simulink model "pothole_test"  (R2025a)
settings: Solver=VariableStepAuto  StartTime=0.0  StopTime=10.0  RelTol=1e-3
model workspace (MAT data in the model file):
  vehicle_car = Simulink.Parameter
  vehicle_car.Complexity = 'real'
  vehicle_car.Dimensions = [0 0]
  vehicle_car.DataType = 'auto'
undefined symbols (not defined in the file or in its folder): Defined, Ego, Lane, User
libraries: roadrunnerscenario x4
settings Model: Creator=Shreyas Hegde  LastModifiedBy=Shreyas Hegde

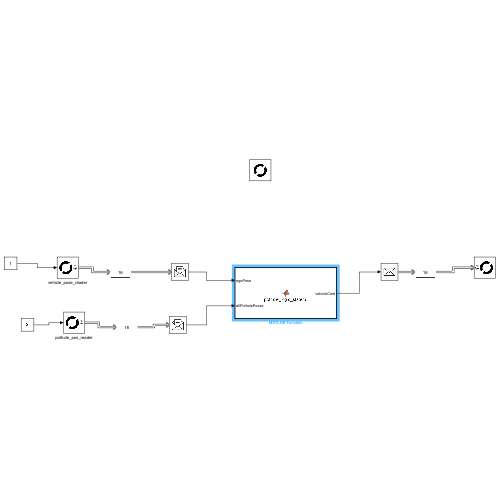
[thumbnail: Simulink's stored preview of the top-level diagram]
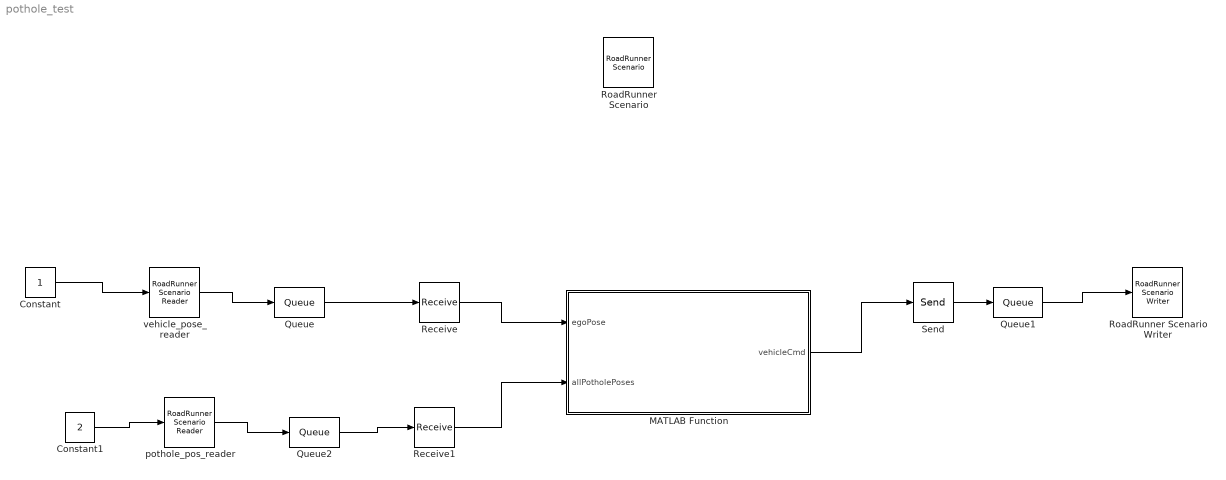
== system pothole_test ==
  Constant : Constant
  Constant1 : Constant  Value=2
  MATLAB Function : MATLAB Function  TreatAsAtomicUnit=on
  Queue : Queue  InputPortMessageModes=m  OutputPortMessageModes=m  OverwriteOldest=on  Capacity=16  QueueType=LIFO
  Queue1 : Queue  InputPortMessageModes=m  OutputPortMessageModes=m  OverwriteOldest=on  Capacity=16  QueueType=LIFO
  Queue2 : Queue  InputPortMessageModes=m  OutputPortMessageModes=m  OverwriteOldest=on  Capacity=16  QueueType=LIFO
  Receive : Receive  InputPortMessageModes=m  UseInternalQueue=off  QueueOverwriting=on  QueueLength=1  QueueType=LIFO
  Receive1 : Receive  InputPortMessageModes=m  UseInternalQueue=off  QueueOverwriting=on  QueueLength=1  QueueType=LIFO
  RoadRunner Scenario : roadrunnerscenario/RoadRunner Scenario  UserDefinedActions={}  UserDefinedEvents={}  PathPoints=500
  RoadRunner Scenario Writer : roadrunnerscenario/RoadRunner Scenario Writer  TopicCategory=Actor  ActorCategory=All Types  EventType=Action Complete  UserDefinedEvent=Event1  VehicleType=Vehicle Pose  TopicType=Actor Pose
  Send : Send  OutputPortMessageModes=m
  pothole_pos_reader : roadrunnerscenario/RoadRunner Scenario Reader  TopicCategory=Actor  ActorCategory=All Types  ActionType=Path Following  EventType=User-Defined  TopicType=Actor Pose  VehicleType=Vehicle Specifications  TrafficSignalType=Traffic Signal Specifications  TrafficSignalControllerType=Traffic Signal Controller Specifications  UserDefinedAction=Action1  UserDefinedEvent=Event1  Filter=Actor ID (provided by input)  AdditionalRelationship=None  SensorTopic=Target Poses  LaneBoundaryOutputTopic=Ego-Lane  SensorID=1  SampleTime=0
  vehicle_pose_reader : roadrunnerscenario/RoadRunner Scenario Reader  TopicCategory=Actor  ActorCategory=All Types  ActionType=Path Following  EventType=User-Defined  TopicType=Actor Pose  VehicleType=Vehicle Specifications  TrafficSignalType=Traffic Signal Specifications  TrafficSignalControllerType=Traffic Signal Controller Specifications  UserDefinedAction=Action1  UserDefinedEvent=Event1  Filter=Actor ID (provided by input)  AdditionalRelationship=None  SensorTopic=Target Poses  LaneBoundaryOutputTopic=Ego-Lane  SensorID=1  SampleTime=0
  wires:
  vehicle_pose_reader/1 -> Queue/1
  Queue/1 -> Receive/1
  Send/1 -> Queue1/1
  Queue1/1 -> RoadRunner Scenario Writer/1
  pothole_pos_reader/1 -> Queue2/1
  Queue2/1 -> Receive1/1
  Receive/1 -> MATLAB Function/1(egoPose)
  Receive1/1 -> MATLAB Function/2(allPotholePoses)
  MATLAB Function/1(vehicleCmd) -> Send/1
  Constant/1 -> vehicle_pose_reader/1
  Constant1/1 -> pothole_pos_reader/1

== matlab function pothole_test/MATLAB Function ==
  data: egoPose input; vehicleCmd output; allPotholePoses input
function vehicleCmd = pothole_logic_stateful(egoPose, allPotholePoses)
% This function uses persistent variables to continuously track the next
% pothole and command the vehicle speed.

% --- Tunable Parameters ---
CRUISING_SPEED = 15;  % m/s (approx 54 km/h)
POTHOLE_SPEED = 5;    % m/s (approx 18 km/h)
ACTION_DISTANCE = 50; % meters

% Use a persistent variable to store the ID of the current target pothole.
persistent targetPotholeID;
if isempty(targetPotholeID)
    targetPotholeID = -1; % Initialize on the first run
end

% Initialize the output command bus to tell Simulink the data type
vehicleCmd = Simulink.Bus.createMATLABStruct('slBusActorCommand');
vehicleCmd.ActorName = "vehicle_car"; % Command is always for our car
vehicleCmd.TargetSpeed = CRUISING_SPEED; % Default to cruising speed

% Exit early if the simulation hasn't provided valid actor data yet
if isempty(egoPose) || egoPose.ActorID == 0
    return;
end

% --- State Machine Logic ---

% 1. Find a new target if we don't currently have one.
if targetPotholeID == -1
    targetPotholeID = findNextPothole(egoPose, allPotholePoses.Poses, -1);
end

% If we still can't find a target (e.g., no potholes left), just cruise.
if targetPotholeID == -1
    return;
end

% 2. Get the current position of our target pothole.
targetPotholePose = struct.empty;
for i = 1:numel(allPotholePoses.Poses)
    if allPotholePoses.Poses(i).ActorID == targetPotholeID
        targetPotholePose = allPotholePoses.Poses(i);
        break;
    end
end

% If our target has vanished for some reason, reset and find a new one next step.
if isempty(targetPotholePose)
    targetPotholeID = -1;
    return;
end

% 3. Decide action based on position relative to the target.
vecToPothole = [targetPotholePose.X - egoPose.X, targetPotholePose.Y - egoPose.Y];
yawAngle = -egoPose.Yaw + pi/2; % Convert RR yaw to standard angle
forwardVec = [cos(yawAngle), sin(yawAngle)];

if dot(vecToPothole, forwardVec) < 0 
    % The pothole is behind us. We've passed it.
    % Find the next closest one, making sure to exclude the one we just passed.
    passedPotholeID = targetPotholeID;
    targetPotholeID = findNextPothole(egoPose, allPotholePoses.Poses, passedPotholeID);
    vehicleCmd.TargetSpeed = CRUISING_SPEED; % Accelerate back to cruising
else
    % The pothole is still in front. Check the distance.
    distToPothole = norm(vecToPothole);
    if distToPothole <= ACTION_DISTANCE
        % We are within the action radius, so slow down.
        vehicleCmd.TargetSpeed = POTHOLE_SPEED;
    else
        % We are approaching but still far away, so keep cruising.
        vehicleCmd.TargetSpeed = CRUISING_SPEED;
    end
end


% --- Local Helper Function to find the closest pothole in front ---
function nextPotholeID = findNextPothole(ego, potholes, excludeID)
    minDist = inf;
    nextPotholeID = -1;
    egoYaw = -ego.Yaw + pi/2;
    egoFwdVec = [cos(egoYaw), sin(egoYaw)];
    
    for k = 1:numel(potholes)
        pothole = potholes(k);
        % Skip invalid actors or the one we want to exclude
        if pothole.ActorID == 0 || pothole.ActorID == excludeID
            continue;
        end
        
        vecTo = [pothole.X - ego.X, pothole.Y - ego.Y];
        
        % Check if the pothole is generally in front of us
        if dot(vecTo, egoFwdVec) > 0
            dist = norm(vecTo);
            if dist < minDist
                minDist = dist;
                nextPotholeID = pothole.ActorID;
            end
        end
    end
end

end
